simulink model "Snake"  (R2016a)
settings: Solver=VariableStepAuto  StartTime=0.0  StopTime=inf  RelTol=1e-3
libraries: simulink_extras x57, Snake_Lib x44, Arithmetic_Operations_Lib x28, Bit_Multiplexers_Lib x10, Bit_Demultiplexers_Lib x10, commutil2 x6, Decoders_Lib x4, Memory_Blocks_Lib x3, dspsnks4 x1, Miscellaneous x1
(part 2 of 2)

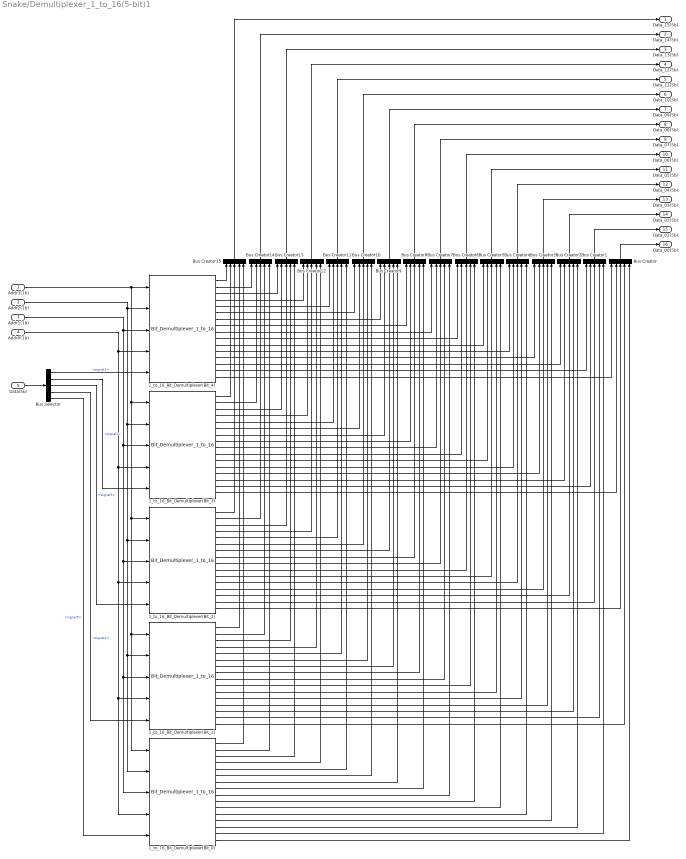
== system Snake/Demultiplexer_1_to_16(5-bit)1 ==
  Addr3(1b) : Inport
  Addr2(1b) : Inport  Port=2
  Addr1(1b) : Inport  Port=3
  Addr0(1b) : Inport  Port=4
  Data(5b) : Inport  Port=5
  1_to_16_Bit_Demultiplexer(Bit_0) : Bit_Demultiplexers_Lib/Bit_Demultiplexers_Lib/Bit_Demultiplexer_1_to_16
  1_to_16_Bit_Demultiplexer(Bit_1) : Bit_Demultiplexers_Lib/Bit_Demultiplexers_Lib/Bit_Demultiplexer_1_to_16
  1_to_16_Bit_Demultiplexer(Bit_2) : Bit_Demultiplexers_Lib/Bit_Demultiplexers_Lib/Bit_Demultiplexer_1_to_16
  1_to_16_Bit_Demultiplexer(Bit_3) : Bit_Demultiplexers_Lib/Bit_Demultiplexers_Lib/Bit_Demultiplexer_1_to_16
  1_to_16_Bit_Demultiplexer(Bit_4) : Bit_Demultiplexers_Lib/Bit_Demultiplexers_Lib/Bit_Demultiplexer_1_to_16
  Bus Creator{,1..15} (16 alike) : BusCreator  Inputs=5
  Bus Selector : BusSelector  OutputSignals=signal1,signal2,signal3,signal4,signal5
  Data_15(5b) : Outport
  Data_14(5b) : Outport  Port=2
  Data_13(5b) : Outport  Port=3
  Data_12(5b) : Outport  Port=4
  Data_11(5b) : Outport  Port=5
  Data_10(5b) : Outport  Port=6
  Data_09(5b) : Outport  Port=7
  Data_08(5b) : Outport  Port=8
  Data_07(5b) : Outport  Port=9
  Data_06(5b) : Outport  Port=10
  Data_05(5b) : Outport  Port=11
  Data_04(5b) : Outport  Port=12
  Data_03(5b) : Outport  Port=13
  Data_02(5b) : Outport  Port=14
  Data_01(5b) : Outport  Port=15
  Data_00(5b) : Outport  Port=16
  wires:
  Bus Selector/4 -> 1_to_16_Bit_Demultiplexer(Bit_1)/5  "<signal4>"
  Bus Selector/5 -> 1_to_16_Bit_Demultiplexer(Bit_0)/5  "<signal5>"
  Bus Selector/3 -> 1_to_16_Bit_Demultiplexer(Bit_2)/5  "<signal3>"
  Bus Selector/2 -> 1_to_16_Bit_Demultiplexer(Bit_3)/5  "<signal2>"
  Bus Selector/1 -> 1_to_16_Bit_Demultiplexer(Bit_4)/5  "<signal1>"
  Bus Creator15/1 -> Data_15(5b)/1
  Bus Creator14/1 -> Data_14(5b)/1
  Bus Creator13/1 -> Data_13(5b)/1
  Bus Creator12/1 -> Data_12(5b)/1
  Bus Creator11/1 -> Data_11(5b)/1
  Bus Creator10/1 -> Data_10(5b)/1
  Bus Creator9/1 -> Data_09(5b)/1
  Bus Creator8/1 -> Data_08(5b)/1
  Bus Creator7/1 -> Data_07(5b)/1
  Bus Creator6/1 -> Data_06(5b)/1
  Bus Creator5/1 -> Data_05(5b)/1
  Bus Creator4/1 -> Data_04(5b)/1
  Bus Creator3/1 -> Data_03(5b)/1
  Bus Creator2/1 -> Data_02(5b)/1
  Bus Creator1/1 -> Data_01(5b)/1
  Bus Creator/1 -> Data_00(5b)/1
  1_to_16_Bit_Demultiplexer(Bit_0)/16 -> Bus Creator/5
  1_to_16_Bit_Demultiplexer(Bit_0)/15 -> Bus Creator1/5
  1_to_16_Bit_Demultiplexer(Bit_0)/14 -> Bus Creator2/5
  1_to_16_Bit_Demultiplexer(Bit_0)/13 -> Bus Creator3/5
  1_to_16_Bit_Demultiplexer(Bit_0)/12 -> Bus Creator4/5
  1_to_16_Bit_Demultiplexer(Bit_0)/11 -> Bus Creator5/5
  1_to_16_Bit_Demultiplexer(Bit_0)/10 -> Bus Creator6/5
  1_to_16_Bit_Demultiplexer(Bit_0)/9 -> Bus Creator7/5
  1_to_16_Bit_Demultiplexer(Bit_0)/8 -> Bus Creator8/5
  1_to_16_Bit_Demultiplexer(Bit_0)/7 -> Bus Creator9/5
  1_to_16_Bit_Demultiplexer(Bit_0)/6 -> Bus Creator10/5
  1_to_16_Bit_Demultiplexer(Bit_0)/5 -> Bus Creator11/5
  1_to_16_Bit_Demultiplexer(Bit_0)/4 -> Bus Creator12/5
  1_to_16_Bit_Demultiplexer(Bit_0)/3 -> Bus Creator13/5
  1_to_16_Bit_Demultiplexer(Bit_0)/2 -> Bus Creator14/5
  1_to_16_Bit_Demultiplexer(Bit_0)/1 -> Bus Creator15/5
  1_to_16_Bit_Demultiplexer(Bit_1)/16 -> Bus Creator/4
  1_to_16_Bit_Demultiplexer(Bit_1)/15 -> Bus Creator1/4
  1_to_16_Bit_Demultiplexer(Bit_1)/14 -> Bus Creator2/4
  1_to_16_Bit_Demultiplexer(Bit_1)/13 -> Bus Creator3/4
  1_to_16_Bit_Demultiplexer(Bit_1)/12 -> Bus Creator4/4
  1_to_16_Bit_Demultiplexer(Bit_1)/11 -> Bus Creator5/4
  1_to_16_Bit_Demultiplexer(Bit_1)/10 -> Bus Creator6/4
  1_to_16_Bit_Demultiplexer(Bit_1)/9 -> Bus Creator7/4
  1_to_16_Bit_Demultiplexer(Bit_1)/8 -> Bus Creator8/4
  1_to_16_Bit_Demultiplexer(Bit_1)/7 -> Bus Creator9/4
  1_to_16_Bit_Demultiplexer(Bit_1)/6 -> Bus Creator10/4
  1_to_16_Bit_Demultiplexer(Bit_1)/5 -> Bus Creator11/4
  1_to_16_Bit_Demultiplexer(Bit_1)/4 -> Bus Creator12/4
  1_to_16_Bit_Demultiplexer(Bit_1)/3 -> Bus Creator13/4
  1_to_16_Bit_Demultiplexer(Bit_1)/2 -> Bus Creator14/4
  1_to_16_Bit_Demultiplexer(Bit_1)/1 -> Bus Creator15/4
  1_to_16_Bit_Demultiplexer(Bit_2)/16 -> Bus Creator/3
  1_to_16_Bit_Demultiplexer(Bit_2)/15 -> Bus Creator1/3
  1_to_16_Bit_Demultiplexer(Bit_2)/14 -> Bus Creator2/3
  1_to_16_Bit_Demultiplexer(Bit_2)/13 -> Bus Creator3/3
  1_to_16_Bit_Demultiplexer(Bit_2)/12 -> Bus Creator4/3
  1_to_16_Bit_Demultiplexer(Bit_2)/11 -> Bus Creator5/3
  1_to_16_Bit_Demultiplexer(Bit_2)/10 -> Bus Creator6/3
  1_to_16_Bit_Demultiplexer(Bit_2)/9 -> Bus Creator7/3
  1_to_16_Bit_Demultiplexer(Bit_2)/8 -> Bus Creator8/3
  1_to_16_Bit_Demultiplexer(Bit_2)/7 -> Bus Creator9/3
  1_to_16_Bit_Demultiplexer(Bit_2)/6 -> Bus Creator10/3
  1_to_16_Bit_Demultiplexer(Bit_2)/5 -> Bus Creator11/3
  1_to_16_Bit_Demultiplexer(Bit_2)/4 -> Bus Creator12/3
  1_to_16_Bit_Demultiplexer(Bit_2)/3 -> Bus Creator13/3
  1_to_16_Bit_Demultiplexer(Bit_2)/2 -> Bus Creator14/3
  1_to_16_Bit_Demultiplexer(Bit_2)/1 -> Bus Creator15/3
  1_to_16_Bit_Demultiplexer(Bit_3)/16 -> Bus Creator/2
  1_to_16_Bit_Demultiplexer(Bit_3)/15 -> Bus Creator1/2
  1_to_16_Bit_Demultiplexer(Bit_3)/14 -> Bus Creator2/2
  1_to_16_Bit_Demultiplexer(Bit_3)/13 -> Bus Creator3/2
  1_to_16_Bit_Demultiplexer(Bit_3)/12 -> Bus Creator4/2
  1_to_16_Bit_Demultiplexer(Bit_3)/11 -> Bus Creator5/2
  1_to_16_Bit_Demultiplexer(Bit_3)/10 -> Bus Creator6/2
  1_to_16_Bit_Demultiplexer(Bit_3)/9 -> Bus Creator7/2
  1_to_16_Bit_Demultiplexer(Bit_3)/8 -> Bus Creator8/2
  1_to_16_Bit_Demultiplexer(Bit_3)/7 -> Bus Creator9/2
  1_to_16_Bit_Demultiplexer(Bit_3)/6 -> Bus Creator10/2
  1_to_16_Bit_Demultiplexer(Bit_3)/5 -> Bus Creator11/2
  1_to_16_Bit_Demultiplexer(Bit_3)/4 -> Bus Creator12/2
  1_to_16_Bit_Demultiplexer(Bit_3)/3 -> Bus Creator13/2
  1_to_16_Bit_Demultiplexer(Bit_3)/2 -> Bus Creator14/2
  1_to_16_Bit_Demultiplexer(Bit_3)/1 -> Bus Creator15/2
  1_to_16_Bit_Demultiplexer(Bit_4)/16 -> Bus Creator/1
  1_to_16_Bit_Demultiplexer(Bit_4)/15 -> Bus Creator1/1
  1_to_16_Bit_Demultiplexer(Bit_4)/14 -> Bus Creator2/1
  1_to_16_Bit_Demultiplexer(Bit_4)/13 -> Bus Creator3/1
  1_to_16_Bit_Demultiplexer(Bit_4)/12 -> Bus Creator4/1
  1_to_16_Bit_Demultiplexer(Bit_4)/11 -> Bus Creator5/1
  1_to_16_Bit_Demultiplexer(Bit_4)/10 -> Bus Creator6/1
  1_to_16_Bit_Demultiplexer(Bit_4)/9 -> Bus Creator7/1
  1_to_16_Bit_Demultiplexer(Bit_4)/8 -> Bus Creator8/1
  1_to_16_Bit_Demultiplexer(Bit_4)/7 -> Bus Creator9/1
  1_to_16_Bit_Demultiplexer(Bit_4)/6 -> Bus Creator10/1
  1_to_16_Bit_Demultiplexer(Bit_4)/5 -> Bus Creator11/1
  1_to_16_Bit_Demultiplexer(Bit_4)/4 -> Bus Creator12/1
  1_to_16_Bit_Demultiplexer(Bit_4)/3 -> Bus Creator13/1
  1_to_16_Bit_Demultiplexer(Bit_4)/2 -> Bus Creator14/1
  1_to_16_Bit_Demultiplexer(Bit_4)/1 -> Bus Creator15/1
  Data(5b)/1 -> Bus Selector/1
  Addr3(1b)/1 -> 1_to_16_Bit_Demultiplexer(Bit_4)/1, 1_to_16_Bit_Demultiplexer(Bit_3)/1, 1_to_16_Bit_Demultiplexer(Bit_2)/1, 1_to_16_Bit_Demultiplexer(Bit_1)/1, 1_to_16_Bit_Demultiplexer(Bit_0)/1
  Addr2(1b)/1 -> 1_to_16_Bit_Demultiplexer(Bit_3)/2, 1_to_16_Bit_Demultiplexer(Bit_2)/2, 1_to_16_Bit_Demultiplexer(Bit_1)/2, 1_to_16_Bit_Demultiplexer(Bit_0)/2, 1_to_16_Bit_Demultiplexer(Bit_4)/2
  Addr1(1b)/1 -> 1_to_16_Bit_Demultiplexer(Bit_3)/3, 1_to_16_Bit_Demultiplexer(Bit_2)/3, 1_to_16_Bit_Demultiplexer(Bit_1)/3, 1_to_16_Bit_Demultiplexer(Bit_0)/3, 1_to_16_Bit_Demultiplexer(Bit_4)/3
  Addr0(1b)/1 -> 1_to_16_Bit_Demultiplexer(Bit_3)/4, 1_to_16_Bit_Demultiplexer(Bit_2)/4, 1_to_16_Bit_Demultiplexer(Bit_1)/4, 1_to_16_Bit_Demultiplexer(Bit_0)/4, 1_to_16_Bit_Demultiplexer(Bit_4)/4

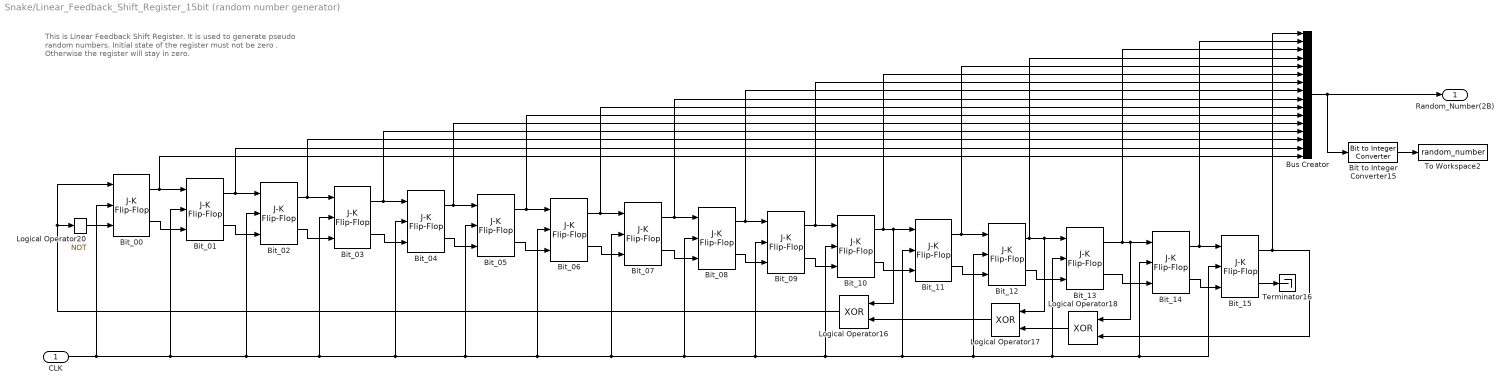
== system Snake/Linear_Feedback_Shift_Register_15bit (random number generator) ==
  note: This is Linear Feedback Shift Register. It is used to generate pseudo random numbers. Initial state of the register must not be zero . Otherwise the register will stay in zero.
  CLK : Inport
  Bit to Integer Converter15 : commutil2/Bit to Integer Converter  nbits=16  bitOrder=MSB first  signedOutputValues=Unsigned  outDtype=uint16  outDtypeSigned=Inherit via internal rule
  Bit_00 : simulink_extras/Flip Flops/J-K Flip-Flop  initial_condition=1
  Bit_01 : simulink_extras/Flip Flops/J-K Flip-Flop  initial_condition=0
  Bit_02 : simulink_extras/Flip Flops/J-K Flip-Flop  initial_condition=0
  Bit_03 : simulink_extras/Flip Flops/J-K Flip-Flop  initial_condition=0
  Bit_04 : simulink_extras/Flip Flops/J-K Flip-Flop  initial_condition=0
  Bit_05 : simulink_extras/Flip Flops/J-K Flip-Flop  initial_condition=0
  Bit_06 : simulink_extras/Flip Flops/J-K Flip-Flop  initial_condition=0
  Bit_07 : simulink_extras/Flip Flops/J-K Flip-Flop  initial_condition=0
  Bit_08 : simulink_extras/Flip Flops/J-K Flip-Flop  initial_condition=0
  Bit_09 : simulink_extras/Flip Flops/J-K Flip-Flop  initial_condition=0
  Bit_{10..15} (6 alike) : simulink_extras/Flip Flops/J-K Flip-Flop  initial_condition=0
  Bus Creator : BusCreator  Inputs=16
  Logical Operator16 : Logic  Operator=XOR  IconShape=distinctive  AllPortsSameDT=off  OutDataTypeStr=boolean
  Logical Operator17 : Logic  Operator=XOR  IconShape=distinctive  AllPortsSameDT=off  OutDataTypeStr=boolean
  Logical Operator18 : Logic  Operator=XOR  IconShape=distinctive  AllPortsSameDT=off  OutDataTypeStr=boolean
  Logical Operator20 : Logic  Operator=NOT  IconShape=distinctive  AllPortsSameDT=off  OutDataTypeStr=boolean
  Terminator16 : Terminator
  To Workspace2 : ToWorkspace  VariableName=random_number  SampleTime=-1
      settings: MaxDataPoints=1  Save2DSignal=2-D array (concatenate along first dimension)
  Random_Number(2B) : Outport
  wires:
  Bit to Integer Converter15/1 -> To Workspace2/1
  Logical Operator20/1 -> Bit_00/3
  Bit_14/2 -> Bit_15/3
  Bit_06/2 -> Bit_07/3
  Bit_04/2 -> Bit_05/3
  Logical Operator18/1 -> Logical Operator17/2
  Logical Operator17/1 -> Logical Operator16/2
  Bit_00/2 -> Bit_01/3
  Logical Operator16/1 -> Logical Operator20/1, Bit_00/1
  Bit_02/2 -> Bit_03/3
  Bit_03/2 -> Bit_04/3
  Bit_01/2 -> Bit_02/3
  Bit_05/2 -> Bit_06/3
  Bit_07/2 -> Bit_08/3
  Bit_09/2 -> Bit_10/3
  Bit_10/2 -> Bit_11/3
  Bit_08/2 -> Bit_09/3
  Bit_13/2 -> Bit_14/3
  Bit_12/2 -> Bit_13/3
  Bit_11/2 -> Bit_12/3
  Bit_00/1 -> Bus Creator/16, Bit_01/1
  CLK/1 -> Bit_00/2, Bit_01/2, Bit_02/2, Bit_03/2, Bit_04/2, Bit_05/2, Bit_06/2, Bit_07/2, Bit_08/2, Bit_09/2, Bit_10/2, Bit_11/2, Bit_12/2, Bit_13/2, Bit_14/2, Bit_15/2
  Bit_15/1 -> Bus Creator/1, Logical Operator18/2
  Bit_15/2 -> Terminator16/1
  Bit_01/1 -> Bus Creator/15, Bit_02/1
  Bit_02/1 -> Bus Creator/14, Bit_03/1
  Bit_03/1 -> Bus Creator/13, Bit_04/1
  Bit_04/1 -> Bus Creator/12, Bit_05/1
  Bit_05/1 -> Bus Creator/11, Bit_06/1
  Bit_06/1 -> Bus Creator/10, Bit_07/1
  Bit_07/1 -> Bus Creator/9, Bit_08/1
  Bit_08/1 -> Bus Creator/8, Bit_09/1
  Bit_09/1 -> Bus Creator/7, Bit_10/1
  Bit_10/1 -> Bus Creator/6, Bit_11/1, Logical Operator16/1
  Bit_12/1 -> Bus Creator/4, Bit_13/1, Logical Operator17/1
  Bit_13/1 -> Bus Creator/3, Bit_14/1, Logical Operator18/1
  Bit_14/1 -> Bus Creator/2, Bit_15/1
  Bit_11/1 -> Bus Creator/5, Bit_12/1
  Bus Creator/1 -> Random_Number(2B)/1, Bit to Integer Converter15/1

== system Snake/Push Button ==

== system Snake/Push Button1 ==

== system Snake/Push Button2 ==

== system Snake/Push Button3 ==

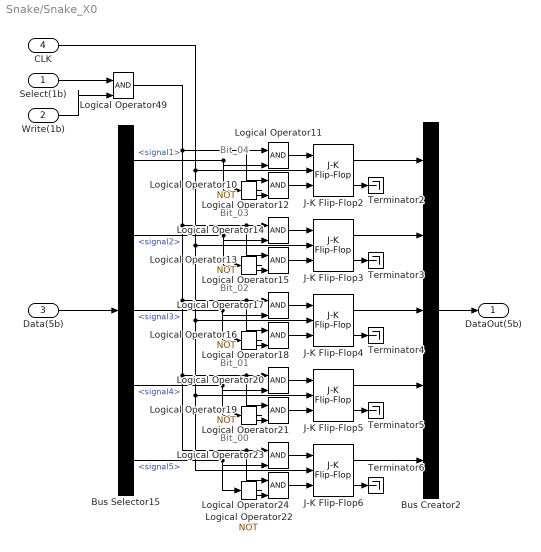
== system Snake/Snake_X0 ==
  note: Bit_04
  note: Bit_03
  note: Bit_02
  note: Bit_01
  note: Bit_00
  Select(1b) : Inport
  Write(1b) : Inport  Port=2
  Data(5b) : Inport  Port=3
  CLK : Inport  Port=4  OutDataTypeStr=double
  Bus Creator2 : BusCreator  Inputs=5
  Bus Selector15 : BusSelector  OutputSignals=signal1,signal2,signal3,signal4,signal5
  J-K Flip-Flop{2..6} (5 alike) : simulink_extras/Flip Flops/J-K Flip-Flop  initial_condition=0
  Logical Operator{10,13,16,19,22} (5 alike) : Logic  Operator=NOT  IconShape=distinctive  AllPortsSameDT=off  OutDataTypeStr=boolean
  Logical Operator{11..12,14..15,17..18,20..21,23..24,49} (11 alike) : Logic  IconShape=distinctive  AllPortsSameDT=off  OutDataTypeStr=boolean
  Terminator{2..6} (5 alike) : Terminator
  DataOut(5b) : Outport
  wires:
  Write(1b)/1 -> Logical Operator49/2
  Select(1b)/1 -> Logical Operator49/1
  Data(5b)/1 -> Bus Selector15/1
  CLK/1 -> J-K Flip-Flop6/2, J-K Flip-Flop5/2, J-K Flip-Flop4/2, J-K Flip-Flop3/2, J-K Flip-Flop2/2
  Logical Operator12/1 -> J-K Flip-Flop2/3
  Logical Operator11/1 -> J-K Flip-Flop2/1
  Logical Operator10/1 -> Logical Operator12/2
  J-K Flip-Flop2/1 -> Bus Creator2/1
  J-K Flip-Flop2/2 -> Terminator2/1
  Bus Selector15/1 -> Logical Operator11/2, Logical Operator10/1  "<signal1>"
  Logical Operator15/1 -> J-K Flip-Flop3/3
  Logical Operator14/1 -> J-K Flip-Flop3/1
  Logical Operator13/1 -> Logical Operator15/2
  J-K Flip-Flop3/1 -> Bus Creator2/2
  J-K Flip-Flop3/2 -> Terminator3/1
  Bus Selector15/2 -> Logical Operator13/1, Logical Operator14/2  "<signal2>"
  Logical Operator18/1 -> J-K Flip-Flop4/3
  Logical Operator17/1 -> J-K Flip-Flop4/1
  Logical Operator16/1 -> Logical Operator18/2
  J-K Flip-Flop4/1 -> Bus Creator2/3
  J-K Flip-Flop4/2 -> Terminator4/1
  Bus Selector15/3 -> Logical Operator16/1, Logical Operator17/2  "<signal3>"
  Logical Operator21/1 -> J-K Flip-Flop5/3
  Logical Operator20/1 -> J-K Flip-Flop5/1
  Logical Operator19/1 -> Logical Operator21/2
  Logical Operator49/1 -> Logical Operator12/1, Logical Operator11/1, Logical Operator15/1, Logical Operator14/1, Logical Operator18/1, Logical Operator17/1, Logical Operator24/1, Logical Operator23/1, Logical Operator21/1, Logical Operator20/1
  J-K Flip-Flop5/1 -> Bus Creator2/4
  J-K Flip-Flop5/2 -> Terminator5/1
  Bus Selector15/4 -> Logical Operator20/2, Logical Operator19/1  "<signal4>"
  Logical Operator24/1 -> J-K Flip-Flop6/3
  Logical Operator23/1 -> J-K Flip-Flop6/1
  Logical Operator22/1 -> Logical Operator24/2
  J-K Flip-Flop6/1 -> Bus Creator2/5
  J-K Flip-Flop6/2 -> Terminator6/1
  Bus Selector15/5 -> Logical Operator23/2, Logical Operator22/1  "<signal5>"
  Bus Creator2/1 -> DataOut(5b)/1

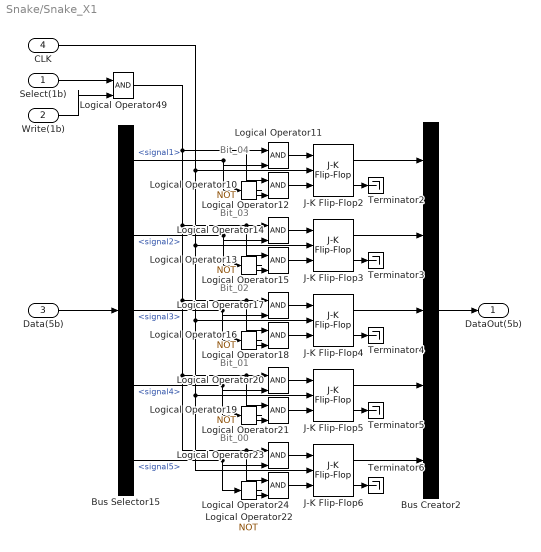
== system Snake/Snake_X1 ==
  note: Bit_04
  note: Bit_03
  note: Bit_02
  note: Bit_01
  note: Bit_00
  Select(1b) : Inport
  Write(1b) : Inport  Port=2
  Data(5b) : Inport  Port=3
  CLK : Inport  Port=4  OutDataTypeStr=double
  Bus Creator2 : BusCreator  Inputs=5
  Bus Selector15 : BusSelector  OutputSignals=signal1,signal2,signal3,signal4,signal5
  J-K Flip-Flop{2..5} (4 alike) : simulink_extras/Flip Flops/J-K Flip-Flop  initial_condition=0
  J-K Flip-Flop6 : simulink_extras/Flip Flops/J-K Flip-Flop  initial_condition=1
  Logical Operator{10,13,16,19,22} (5 alike) : Logic  Operator=NOT  IconShape=distinctive  AllPortsSameDT=off  OutDataTypeStr=boolean
  Logical Operator{11..12,14..15,17..18,20..21,23..24,49} (11 alike) : Logic  IconShape=distinctive  AllPortsSameDT=off  OutDataTypeStr=boolean
  Terminator{2..6} (5 alike) : Terminator
  DataOut(5b) : Outport
  wires:
  Write(1b)/1 -> Logical Operator49/2
  Select(1b)/1 -> Logical Operator49/1
  Data(5b)/1 -> Bus Selector15/1
  CLK/1 -> J-K Flip-Flop6/2, J-K Flip-Flop5/2, J-K Flip-Flop4/2, J-K Flip-Flop3/2, J-K Flip-Flop2/2
  Logical Operator12/1 -> J-K Flip-Flop2/3
  Logical Operator11/1 -> J-K Flip-Flop2/1
  Logical Operator10/1 -> Logical Operator12/2
  J-K Flip-Flop2/1 -> Bus Creator2/1
  J-K Flip-Flop2/2 -> Terminator2/1
  Bus Selector15/1 -> Logical Operator11/2, Logical Operator10/1  "<signal1>"
  Logical Operator15/1 -> J-K Flip-Flop3/3
  Logical Operator14/1 -> J-K Flip-Flop3/1
  Logical Operator13/1 -> Logical Operator15/2
  J-K Flip-Flop3/1 -> Bus Creator2/2
  J-K Flip-Flop3/2 -> Terminator3/1
  Bus Selector15/2 -> Logical Operator13/1, Logical Operator14/2  "<signal2>"
  Logical Operator18/1 -> J-K Flip-Flop4/3
  Logical Operator17/1 -> J-K Flip-Flop4/1
  Logical Operator16/1 -> Logical Operator18/2
  J-K Flip-Flop4/1 -> Bus Creator2/3
  J-K Flip-Flop4/2 -> Terminator4/1
  Bus Selector15/3 -> Logical Operator16/1, Logical Operator17/2  "<signal3>"
  Logical Operator21/1 -> J-K Flip-Flop5/3
  Logical Operator20/1 -> J-K Flip-Flop5/1
  Logical Operator19/1 -> Logical Operator21/2
  Logical Operator49/1 -> Logical Operator12/1, Logical Operator11/1, Logical Operator15/1, Logical Operator14/1, Logical Operator18/1, Logical Operator17/1, Logical Operator24/1, Logical Operator23/1, Logical Operator21/1, Logical Operator20/1
  J-K Flip-Flop5/1 -> Bus Creator2/4
  J-K Flip-Flop5/2 -> Terminator5/1
  Bus Selector15/4 -> Logical Operator20/2, Logical Operator19/1  "<signal4>"
  Logical Operator24/1 -> J-K Flip-Flop6/3
  Logical Operator23/1 -> J-K Flip-Flop6/1
  Logical Operator22/1 -> Logical Operator24/2
  J-K Flip-Flop6/1 -> Bus Creator2/5
  J-K Flip-Flop6/2 -> Terminator6/1
  Bus Selector15/5 -> Logical Operator23/2, Logical Operator22/1  "<signal5>"
  Bus Creator2/1 -> DataOut(5b)/1

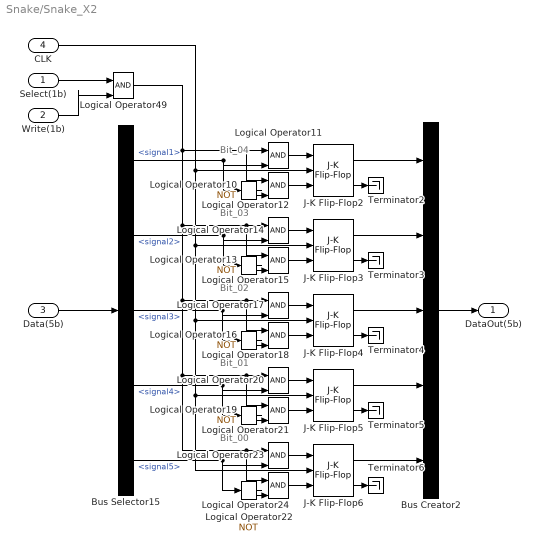
== system Snake/Snake_X2 ==
  note: Bit_04
  note: Bit_03
  note: Bit_02
  note: Bit_01
  note: Bit_00
  Select(1b) : Inport
  Write(1b) : Inport  Port=2
  Data(5b) : Inport  Port=3
  CLK : Inport  Port=4  OutDataTypeStr=double
  Bus Creator2 : BusCreator  Inputs=5
  Bus Selector15 : BusSelector  OutputSignals=signal1,signal2,signal3,signal4,signal5
  J-K Flip-Flop{2..4,6} (4 alike) : simulink_extras/Flip Flops/J-K Flip-Flop  initial_condition=0
  J-K Flip-Flop5 : simulink_extras/Flip Flops/J-K Flip-Flop  initial_condition=1
  Logical Operator{10,13,16,19,22} (5 alike) : Logic  Operator=NOT  IconShape=distinctive  AllPortsSameDT=off  OutDataTypeStr=boolean
  Logical Operator{11..12,14..15,17..18,20..21,23..24,49} (11 alike) : Logic  IconShape=distinctive  AllPortsSameDT=off  OutDataTypeStr=boolean
  Terminator{2..6} (5 alike) : Terminator
  DataOut(5b) : Outport
  wires:
  Write(1b)/1 -> Logical Operator49/2
  Select(1b)/1 -> Logical Operator49/1
  Data(5b)/1 -> Bus Selector15/1
  CLK/1 -> J-K Flip-Flop6/2, J-K Flip-Flop5/2, J-K Flip-Flop4/2, J-K Flip-Flop3/2, J-K Flip-Flop2/2
  Logical Operator12/1 -> J-K Flip-Flop2/3
  Logical Operator11/1 -> J-K Flip-Flop2/1
  Logical Operator10/1 -> Logical Operator12/2
  J-K Flip-Flop2/1 -> Bus Creator2/1
  J-K Flip-Flop2/2 -> Terminator2/1
  Bus Selector15/1 -> Logical Operator11/2, Logical Operator10/1  "<signal1>"
  Logical Operator15/1 -> J-K Flip-Flop3/3
  Logical Operator14/1 -> J-K Flip-Flop3/1
  Logical Operator13/1 -> Logical Operator15/2
  J-K Flip-Flop3/1 -> Bus Creator2/2
  J-K Flip-Flop3/2 -> Terminator3/1
  Bus Selector15/2 -> Logical Operator13/1, Logical Operator14/2  "<signal2>"
  Logical Operator18/1 -> J-K Flip-Flop4/3
  Logical Operator17/1 -> J-K Flip-Flop4/1
  Logical Operator16/1 -> Logical Operator18/2
  J-K Flip-Flop4/1 -> Bus Creator2/3
  J-K Flip-Flop4/2 -> Terminator4/1
  Bus Selector15/3 -> Logical Operator16/1, Logical Operator17/2  "<signal3>"
  Logical Operator21/1 -> J-K Flip-Flop5/3
  Logical Operator20/1 -> J-K Flip-Flop5/1
  Logical Operator19/1 -> Logical Operator21/2
  Logical Operator49/1 -> Logical Operator12/1, Logical Operator11/1, Logical Operator15/1, Logical Operator14/1, Logical Operator18/1, Logical Operator17/1, Logical Operator24/1, Logical Operator23/1, Logical Operator21/1, Logical Operator20/1
  J-K Flip-Flop5/1 -> Bus Creator2/4
  J-K Flip-Flop5/2 -> Terminator5/1
  Bus Selector15/4 -> Logical Operator20/2, Logical Operator19/1  "<signal4>"
  Logical Operator24/1 -> J-K Flip-Flop6/3
  Logical Operator23/1 -> J-K Flip-Flop6/1
  Logical Operator22/1 -> Logical Operator24/2
  J-K Flip-Flop6/1 -> Bus Creator2/5
  J-K Flip-Flop6/2 -> Terminator6/1
  Bus Selector15/5 -> Logical Operator23/2, Logical Operator22/1  "<signal5>"
  Bus Creator2/1 -> DataOut(5b)/1

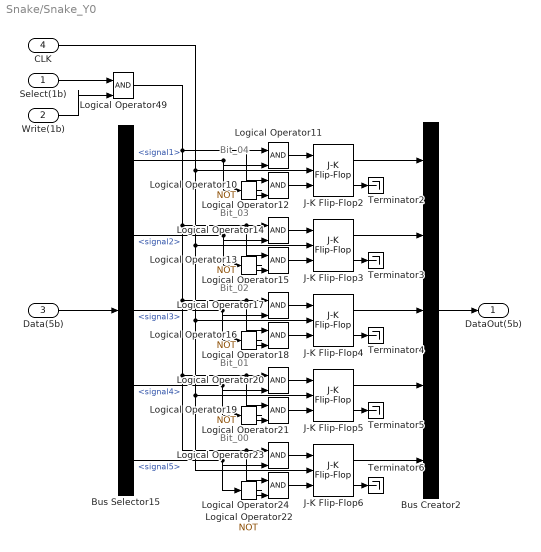
== system Snake/Snake_Y0 ==
  note: Bit_04
  note: Bit_03
  note: Bit_02
  note: Bit_01
  note: Bit_00
  Select(1b) : Inport
  Write(1b) : Inport  Port=2
  Data(5b) : Inport  Port=3
  CLK : Inport  Port=4  OutDataTypeStr=double
  Bus Creator2 : BusCreator  Inputs=5
  Bus Selector15 : BusSelector  OutputSignals=signal1,signal2,signal3,signal4,signal5
  J-K Flip-Flop{2..5} (4 alike) : simulink_extras/Flip Flops/J-K Flip-Flop  initial_condition=0
  J-K Flip-Flop6 : simulink_extras/Flip Flops/J-K Flip-Flop  initial_condition=1
  Logical Operator{10,13,16,19,22} (5 alike) : Logic  Operator=NOT  IconShape=distinctive  AllPortsSameDT=off  OutDataTypeStr=boolean
  Logical Operator{11..12,14..15,17..18,20..21,23..24,49} (11 alike) : Logic  IconShape=distinctive  AllPortsSameDT=off  OutDataTypeStr=boolean
  Terminator{2..6} (5 alike) : Terminator
  DataOut(5b) : Outport
  wires:
  Write(1b)/1 -> Logical Operator49/2
  Select(1b)/1 -> Logical Operator49/1
  Data(5b)/1 -> Bus Selector15/1
  CLK/1 -> J-K Flip-Flop6/2, J-K Flip-Flop5/2, J-K Flip-Flop4/2, J-K Flip-Flop3/2, J-K Flip-Flop2/2
  Logical Operator12/1 -> J-K Flip-Flop2/3
  Logical Operator11/1 -> J-K Flip-Flop2/1
  Logical Operator10/1 -> Logical Operator12/2
  J-K Flip-Flop2/1 -> Bus Creator2/1
  J-K Flip-Flop2/2 -> Terminator2/1
  Bus Selector15/1 -> Logical Operator11/2, Logical Operator10/1  "<signal1>"
  Logical Operator15/1 -> J-K Flip-Flop3/3
  Logical Operator14/1 -> J-K Flip-Flop3/1
  Logical Operator13/1 -> Logical Operator15/2
  J-K Flip-Flop3/1 -> Bus Creator2/2
  J-K Flip-Flop3/2 -> Terminator3/1
  Bus Selector15/2 -> Logical Operator13/1, Logical Operator14/2  "<signal2>"
  Logical Operator18/1 -> J-K Flip-Flop4/3
  Logical Operator17/1 -> J-K Flip-Flop4/1
  Logical Operator16/1 -> Logical Operator18/2
  J-K Flip-Flop4/1 -> Bus Creator2/3
  J-K Flip-Flop4/2 -> Terminator4/1
  Bus Selector15/3 -> Logical Operator16/1, Logical Operator17/2  "<signal3>"
  Logical Operator21/1 -> J-K Flip-Flop5/3
  Logical Operator20/1 -> J-K Flip-Flop5/1
  Logical Operator19/1 -> Logical Operator21/2
  Logical Operator49/1 -> Logical Operator12/1, Logical Operator11/1, Logical Operator15/1, Logical Operator14/1, Logical Operator18/1, Logical Operator17/1, Logical Operator24/1, Logical Operator23/1, Logical Operator21/1, Logical Operator20/1
  J-K Flip-Flop5/1 -> Bus Creator2/4
  J-K Flip-Flop5/2 -> Terminator5/1
  Bus Selector15/4 -> Logical Operator20/2, Logical Operator19/1  "<signal4>"
  Logical Operator24/1 -> J-K Flip-Flop6/3
  Logical Operator23/1 -> J-K Flip-Flop6/1
  Logical Operator22/1 -> Logical Operator24/2
  J-K Flip-Flop6/1 -> Bus Creator2/5
  J-K Flip-Flop6/2 -> Terminator6/1
  Bus Selector15/5 -> Logical Operator23/2, Logical Operator22/1  "<signal5>"
  Bus Creator2/1 -> DataOut(5b)/1

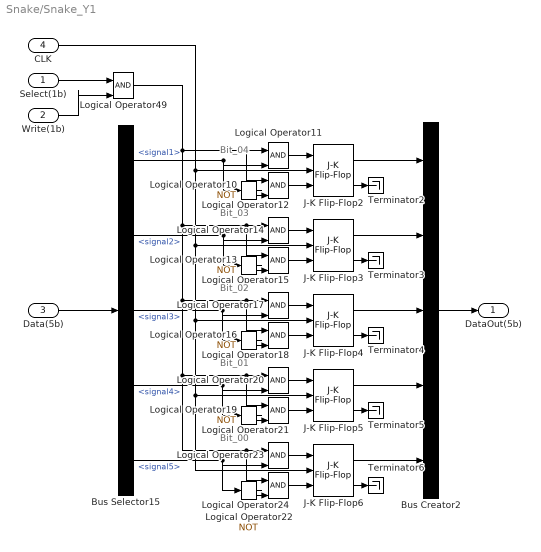
== system Snake/Snake_Y1 ==
  note: Bit_04
  note: Bit_03
  note: Bit_02
  note: Bit_01
  note: Bit_00
  Select(1b) : Inport
  Write(1b) : Inport  Port=2
  Data(5b) : Inport  Port=3
  CLK : Inport  Port=4  OutDataTypeStr=double
  Bus Creator2 : BusCreator  Inputs=5
  Bus Selector15 : BusSelector  OutputSignals=signal1,signal2,signal3,signal4,signal5
  J-K Flip-Flop{2..5} (4 alike) : simulink_extras/Flip Flops/J-K Flip-Flop  initial_condition=0
  J-K Flip-Flop6 : simulink_extras/Flip Flops/J-K Flip-Flop  initial_condition=1
  Logical Operator{10,13,16,19,22} (5 alike) : Logic  Operator=NOT  IconShape=distinctive  AllPortsSameDT=off  OutDataTypeStr=boolean
  Logical Operator{11..12,14..15,17..18,20..21,23..24,49} (11 alike) : Logic  IconShape=distinctive  AllPortsSameDT=off  OutDataTypeStr=boolean
  Terminator{2..6} (5 alike) : Terminator
  DataOut(5b) : Outport
  wires:
  Write(1b)/1 -> Logical Operator49/2
  Select(1b)/1 -> Logical Operator49/1
  Data(5b)/1 -> Bus Selector15/1
  CLK/1 -> J-K Flip-Flop6/2, J-K Flip-Flop5/2, J-K Flip-Flop4/2, J-K Flip-Flop3/2, J-K Flip-Flop2/2
  Logical Operator12/1 -> J-K Flip-Flop2/3
  Logical Operator11/1 -> J-K Flip-Flop2/1
  Logical Operator10/1 -> Logical Operator12/2
  J-K Flip-Flop2/1 -> Bus Creator2/1
  J-K Flip-Flop2/2 -> Terminator2/1
  Bus Selector15/1 -> Logical Operator11/2, Logical Operator10/1  "<signal1>"
  Logical Operator15/1 -> J-K Flip-Flop3/3
  Logical Operator14/1 -> J-K Flip-Flop3/1
  Logical Operator13/1 -> Logical Operator15/2
  J-K Flip-Flop3/1 -> Bus Creator2/2
  J-K Flip-Flop3/2 -> Terminator3/1
  Bus Selector15/2 -> Logical Operator13/1, Logical Operator14/2  "<signal2>"
  Logical Operator18/1 -> J-K Flip-Flop4/3
  Logical Operator17/1 -> J-K Flip-Flop4/1
  Logical Operator16/1 -> Logical Operator18/2
  J-K Flip-Flop4/1 -> Bus Creator2/3
  J-K Flip-Flop4/2 -> Terminator4/1
  Bus Selector15/3 -> Logical Operator16/1, Logical Operator17/2  "<signal3>"
  Logical Operator21/1 -> J-K Flip-Flop5/3
  Logical Operator20/1 -> J-K Flip-Flop5/1
  Logical Operator19/1 -> Logical Operator21/2
  Logical Operator49/1 -> Logical Operator12/1, Logical Operator11/1, Logical Operator15/1, Logical Operator14/1, Logical Operator18/1, Logical Operator17/1, Logical Operator24/1, Logical Operator23/1, Logical Operator21/1, Logical Operator20/1
  J-K Flip-Flop5/1 -> Bus Creator2/4
  J-K Flip-Flop5/2 -> Terminator5/1
  Bus Selector15/4 -> Logical Operator20/2, Logical Operator19/1  "<signal4>"
  Logical Operator24/1 -> J-K Flip-Flop6/3
  Logical Operator23/1 -> J-K Flip-Flop6/1
  Logical Operator22/1 -> Logical Operator24/2
  J-K Flip-Flop6/1 -> Bus Creator2/5
  J-K Flip-Flop6/2 -> Terminator6/1
  Bus Selector15/5 -> Logical Operator23/2, Logical Operator22/1  "<signal5>"
  Bus Creator2/1 -> DataOut(5b)/1

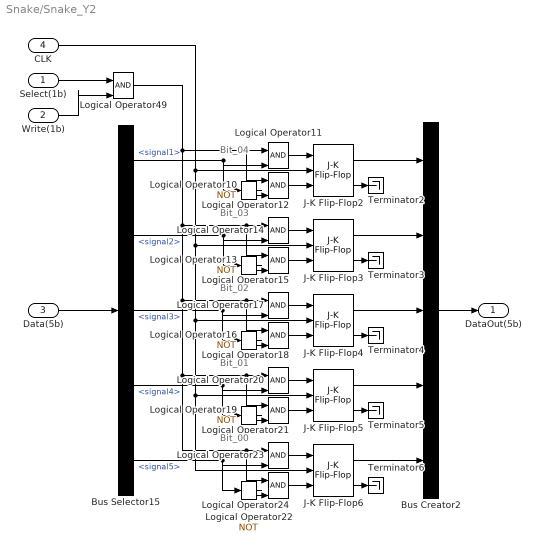
== system Snake/Snake_Y2 ==
  note: Bit_04
  note: Bit_03
  note: Bit_02
  note: Bit_01
  note: Bit_00
  Select(1b) : Inport
  Write(1b) : Inport  Port=2
  Data(5b) : Inport  Port=3
  CLK : Inport  Port=4  OutDataTypeStr=double
  Bus Creator2 : BusCreator  Inputs=5
  Bus Selector15 : BusSelector  OutputSignals=signal1,signal2,signal3,signal4,signal5
  J-K Flip-Flop{2..5} (4 alike) : simulink_extras/Flip Flops/J-K Flip-Flop  initial_condition=0
  J-K Flip-Flop6 : simulink_extras/Flip Flops/J-K Flip-Flop  initial_condition=1
  Logical Operator{10,13,16,19,22} (5 alike) : Logic  Operator=NOT  IconShape=distinctive  AllPortsSameDT=off  OutDataTypeStr=boolean
  Logical Operator{11..12,14..15,17..18,20..21,23..24,49} (11 alike) : Logic  IconShape=distinctive  AllPortsSameDT=off  OutDataTypeStr=boolean
  Terminator{2..6} (5 alike) : Terminator
  DataOut(5b) : Outport
  wires:
  Write(1b)/1 -> Logical Operator49/2
  Select(1b)/1 -> Logical Operator49/1
  Data(5b)/1 -> Bus Selector15/1
  CLK/1 -> J-K Flip-Flop6/2, J-K Flip-Flop5/2, J-K Flip-Flop4/2, J-K Flip-Flop3/2, J-K Flip-Flop2/2
  Logical Operator12/1 -> J-K Flip-Flop2/3
  Logical Operator11/1 -> J-K Flip-Flop2/1
  Logical Operator10/1 -> Logical Operator12/2
  J-K Flip-Flop2/1 -> Bus Creator2/1
  J-K Flip-Flop2/2 -> Terminator2/1
  Bus Selector15/1 -> Logical Operator11/2, Logical Operator10/1  "<signal1>"
  Logical Operator15/1 -> J-K Flip-Flop3/3
  Logical Operator14/1 -> J-K Flip-Flop3/1
  Logical Operator13/1 -> Logical Operator15/2
  J-K Flip-Flop3/1 -> Bus Creator2/2
  J-K Flip-Flop3/2 -> Terminator3/1
  Bus Selector15/2 -> Logical Operator13/1, Logical Operator14/2  "<signal2>"
  Logical Operator18/1 -> J-K Flip-Flop4/3
  Logical Operator17/1 -> J-K Flip-Flop4/1
  Logical Operator16/1 -> Logical Operator18/2
  J-K Flip-Flop4/1 -> Bus Creator2/3
  J-K Flip-Flop4/2 -> Terminator4/1
  Bus Selector15/3 -> Logical Operator16/1, Logical Operator17/2  "<signal3>"
  Logical Operator21/1 -> J-K Flip-Flop5/3
  Logical Operator20/1 -> J-K Flip-Flop5/1
  Logical Operator19/1 -> Logical Operator21/2
  Logical Operator49/1 -> Logical Operator12/1, Logical Operator11/1, Logical Operator15/1, Logical Operator14/1, Logical Operator18/1, Logical Operator17/1, Logical Operator24/1, Logical Operator23/1, Logical Operator21/1, Logical Operator20/1
  J-K Flip-Flop5/1 -> Bus Creator2/4
  J-K Flip-Flop5/2 -> Terminator5/1
  Bus Selector15/4 -> Logical Operator20/2, Logical Operator19/1  "<signal4>"
  Logical Operator24/1 -> J-K Flip-Flop6/3
  Logical Operator23/1 -> J-K Flip-Flop6/1
  Logical Operator22/1 -> Logical Operator24/2
  J-K Flip-Flop6/1 -> Bus Creator2/5
  J-K Flip-Flop6/2 -> Terminator6/1
  Bus Selector15/5 -> Logical Operator23/2, Logical Operator22/1  "<signal5>"
  Bus Creator2/1 -> DataOut(5b)/1

== system Snake/Toggle Switch ==

== system Snake/Toggle Switch1 ==

== system Snake/Toggle Switch2 ==

== system Snake/Toggle Switch3 ==

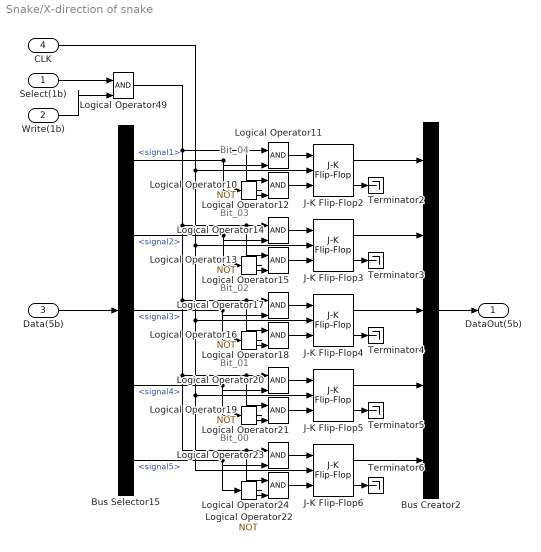
== system Snake/X-direction of snake ==
  note: Bit_04
  note: Bit_03
  note: Bit_02
  note: Bit_01
  note: Bit_00
  Select(1b) : Inport
  Write(1b) : Inport  Port=2
  Data(5b) : Inport  Port=3
  CLK : Inport  Port=4  OutDataTypeStr=double
  Bus Creator2 : BusCreator  Inputs=5
  Bus Selector15 : BusSelector  OutputSignals=signal1,signal2,signal3,signal4,signal5
  J-K Flip-Flop{2..5} (4 alike) : simulink_extras/Flip Flops/J-K Flip-Flop  initial_condition=0
  J-K Flip-Flop6 : simulink_extras/Flip Flops/J-K Flip-Flop  initial_condition=1
  Logical Operator{10,13,16,19,22} (5 alike) : Logic  Operator=NOT  IconShape=distinctive  AllPortsSameDT=off  OutDataTypeStr=boolean
  Logical Operator{11..12,14..15,17..18,20..21,23..24,49} (11 alike) : Logic  IconShape=distinctive  AllPortsSameDT=off  OutDataTypeStr=boolean
  Terminator{2..6} (5 alike) : Terminator
  DataOut(5b) : Outport
  wires:
  Write(1b)/1 -> Logical Operator49/2
  Select(1b)/1 -> Logical Operator49/1
  Data(5b)/1 -> Bus Selector15/1
  CLK/1 -> J-K Flip-Flop6/2, J-K Flip-Flop5/2, J-K Flip-Flop4/2, J-K Flip-Flop3/2, J-K Flip-Flop2/2
  Logical Operator12/1 -> J-K Flip-Flop2/3
  Logical Operator11/1 -> J-K Flip-Flop2/1
  Logical Operator10/1 -> Logical Operator12/2
  J-K Flip-Flop2/1 -> Bus Creator2/1
  J-K Flip-Flop2/2 -> Terminator2/1
  Bus Selector15/1 -> Logical Operator11/2, Logical Operator10/1  "<signal1>"
  Logical Operator15/1 -> J-K Flip-Flop3/3
  Logical Operator14/1 -> J-K Flip-Flop3/1
  Logical Operator13/1 -> Logical Operator15/2
  J-K Flip-Flop3/1 -> Bus Creator2/2
  J-K Flip-Flop3/2 -> Terminator3/1
  Bus Selector15/2 -> Logical Operator13/1, Logical Operator14/2  "<signal2>"
  Logical Operator18/1 -> J-K Flip-Flop4/3
  Logical Operator17/1 -> J-K Flip-Flop4/1
  Logical Operator16/1 -> Logical Operator18/2
  J-K Flip-Flop4/1 -> Bus Creator2/3
  J-K Flip-Flop4/2 -> Terminator4/1
  Bus Selector15/3 -> Logical Operator16/1, Logical Operator17/2  "<signal3>"
  Logical Operator21/1 -> J-K Flip-Flop5/3
  Logical Operator20/1 -> J-K Flip-Flop5/1
  Logical Operator19/1 -> Logical Operator21/2
  Logical Operator49/1 -> Logical Operator12/1, Logical Operator11/1, Logical Operator15/1, Logical Operator14/1, Logical Operator18/1, Logical Operator17/1, Logical Operator24/1, Logical Operator23/1, Logical Operator21/1, Logical Operator20/1
  J-K Flip-Flop5/1 -> Bus Creator2/4
  J-K Flip-Flop5/2 -> Terminator5/1
  Bus Selector15/4 -> Logical Operator20/2, Logical Operator19/1  "<signal4>"
  Logical Operator24/1 -> J-K Flip-Flop6/3
  Logical Operator23/1 -> J-K Flip-Flop6/1
  Logical Operator22/1 -> Logical Operator24/2
  J-K Flip-Flop6/1 -> Bus Creator2/5
  J-K Flip-Flop6/2 -> Terminator6/1
  Bus Selector15/5 -> Logical Operator23/2, Logical Operator22/1  "<signal5>"
  Bus Creator2/1 -> DataOut(5b)/1

== system Snake/uint_to_bus(byte)1 ==
  In(5b) : Inport
  Bus Creator : BusCreator  Inputs=5
  Demux2 : Demux  Outputs=5
  Integer to Bit Converter2 : commutil2/Integer to Bit Converter  nbits=5  signedInputValues=Signed  bitOrder=MSB first  outDtype=boolean
  Out(5b) : Outport
  wires:
  In(5b)/1 -> Integer to Bit Converter2/1
  Bus Creator/1 -> Out(5b)/1
  Integer to Bit Converter2/1 -> Demux2/1
  Demux2/1 -> Bus Creator/1
  Demux2/2 -> Bus Creator/2
  Demux2/3 -> Bus Creator/3
  Demux2/4 -> Bus Creator/4
  Demux2/5 -> Bus Creator/5

== system Snake/uint_to_bus(byte)4 ==
  In(5b) : Inport
  Bus Creator : BusCreator  Inputs=5
  Demux2 : Demux  Outputs=5
  Integer to Bit Converter2 : commutil2/Integer to Bit Converter  nbits=5  signedInputValues=Signed  bitOrder=MSB first  outDtype=boolean
  Out(5b) : Outport
  wires:
  In(5b)/1 -> Integer to Bit Converter2/1
  Bus Creator/1 -> Out(5b)/1
  Integer to Bit Converter2/1 -> Demux2/1
  Demux2/1 -> Bus Creator/1
  Demux2/2 -> Bus Creator/2
  Demux2/3 -> Bus Creator/3
  Demux2/4 -> Bus Creator/4
  Demux2/5 -> Bus Creator/5

== matlab function Snake/MATLAB Function ==
  data: cnt input; Framebuffer output uint32 size=[24 16]; x input; y input
function Framebuffer = Video(cnt, x, y)
%     persistent cnt;
     persistent buffer;
%     persistent Framebuffer;

    SCREEN_MAX_X = 16;
    SCREEN_MAX_Y = 24;

    if isempty(buffer)
        buffer = zeros(SCREEN_MAX_Y, SCREEN_MAX_X, 'uint32');
    end

%     if isempty(cnt)
%         cnt = 0;
%     end
    
%     Framebuffer = zeros(SCREEN_MAX_Y, SCREEN_MAX_X, 'uint32');

%     if (cnt >= 15)
%         cnt = 0;
%     else
%         cnt = cnt + 1;
%     end
    
    % Clear buffer (delete snake).
    if (0 == cnt)
        buffer = zeros(SCREEN_MAX_Y, SCREEN_MAX_X, 'uint32');
    end
    
    switch (x)
        case     1,  x = uint32(1);
        case     2,  x = uint32(2);
        case     4,  x = uint32(3);
        case     8,  x = uint32(4);
        case    16,  x = uint32(5);
        case    32,  x = uint32(6);
        case    64,  x = uint32(7);
        case   128,  x = uint32(8);
        case   256,  x = uint32(9);
        case   512,  x = uint32(10);
        case  1024,  x = uint32(11);
        case  2048,  x = uint32(12);
        case  4096,  x = uint32(13);
        case  8192,  x = uint32(14);
        case 16384,  x = uint32(15);
        case 32768,  x = uint32(16);
    end

    switch (y)
        case       1,  y = uint32(1);
        case       2,  y = uint32(2);
        case       4,  y = uint32(3);
        case       8,  y = uint32(4);
        case      16,  y = uint32(5);
        case      32,  y = uint32(6);
        case      64,  y = uint32(7);
        case     128,  y = uint32(8);
        case     256,  y = uint32(9);
        case     512,  y = uint32(10);
        case    1024,  y = uint32(11);
        case    2048,  y = uint32(12);
        case    4096,  y = uint32(13);
        case    8192,  y = uint32(14);
        case   16384,  y = uint32(15);
        case   32768,  y = uint32(16);
        case   65536,  y = uint32(17);
        case  131072,  y = uint32(18);
        case  262144,  y = uint32(19);
        case  524288,  y = uint32(20);
        case 1048576,  y = uint32(21);
        case 2097152,  y = uint32(22);
        case 4194304,  y = uint32(23);
        case 8388608,  y = uint32(24);
    end

    buffer(y, x) = 1;
    Framebuffer = buffer;
end
